simulink model "SpringiLQR3discrete"  (R2020b)
settings: Solver=FixedStepDiscrete  StartTime=0.0  StopTime=100  FixedStep=0.001  RelTol=1e-3
values from neighbouring files (symbols this model uses):
  A_e = full(kron(Ad, speye(2)))    [SringiLQR2discrete.m]    (also in SringiLQR3discrete.m; mpcgains.m = eye(n1+m1,n1+m1))
  B_e = full(kron(Bd, speye(2)))    [SringiLQR2discrete.m]    (also in SringiLQR3discrete.m; mpcgains.m = zeros(n1+m1,n_in))
  C_e = eye(4)    [SringiLQR2discrete.m]    (also in SringiLQR3discrete.m; mpcgains.m = zeros(m1,n1+m1))
  D_e = zeros(c1,b2)    [SringiLQR2discrete.m]    (also in SringiLQR3discrete.m)
  Dd = 0    [extmodel.m]
  Q = [1 0 0; 0 1 0; 0 0 10]    [LQR.m]    (also in NonlinearVehicleLQR.m = eye(3)*10; NonlinearVehicleiLQR.m = eye(3)*10; SringiLQR.m = [1 0; 0 1]*1; SringiLQR2.m = [1 0; 0 1]*1)
  Qf = eye(3)    [LQR.m]    (also in NonlinearVehicleLQR.m; NonlinearVehicleiLQR.m; SringiLQR.m = [1 0; 0 1]; SringiLQR2.m = [1 0; 0 1])
  R = eye(2)*10^-4    [LQR.m]    (also in NonlinearVehicleLQR.m = eye(2)*10^-2; NonlinearVehicleiLQR.m = eye(2)*10^-2; SringiLQR.m = eye(1)*1e-2; SringiLQR2.m = eye(1)*1e-2)
undefined symbols (not defined in the file or in its folder): Ad, Bd, Cd
libraries: pid_lib x1
settings Model: Creator=iris  LastModifiedBy=iris
settings DebuggingCC: SFMachineParentedDataDiag=error

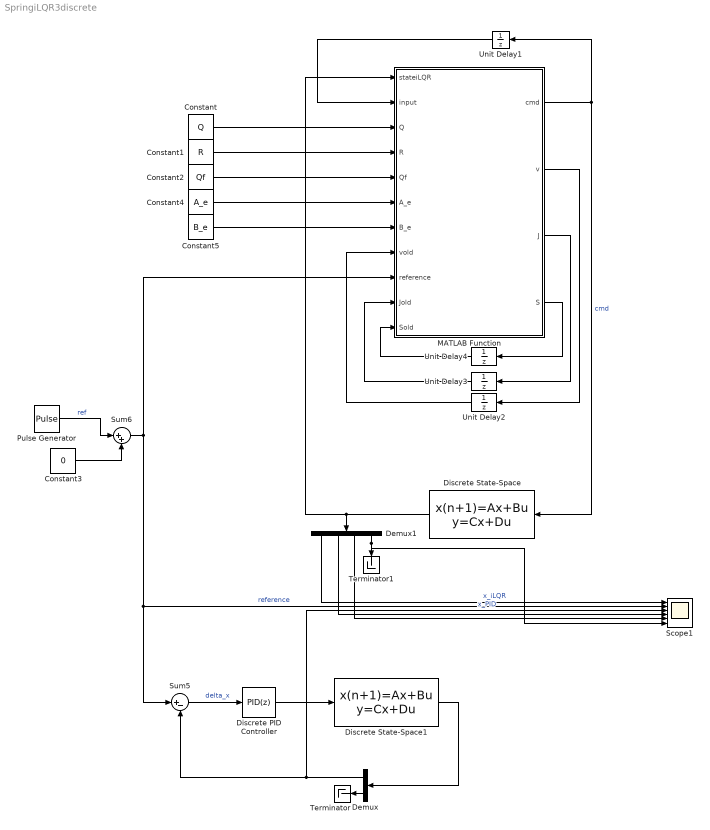
== system SpringiLQR3discrete ==
  Constant : Constant  Value=Q
  Constant1 : Constant  Value=R
  Constant2 : Constant  Value=Qf
  Constant3 : Constant  Value=0
  Constant4 : Constant  Value=A_e
  Constant5 : Constant  Value=B_e
  Demux : Demux  Outputs=2
  Demux1 : Demux
  Discrete PID Controller : pid_lib/PID Controller  Controller=PID  Form=Parallel  TimeDomain=Discrete-time  UseExternalTs=off  SampleTime=-1  IntegratorMethod=Forward Euler  FilterMethod=Forward Euler  ControllerParametersSource=internal  P=0.1  I=0  D=1  UseFilter=on  N=100  TunerSelectOption=Transfer Function Based (PID Tuner App)  InitialConditionSource=internal  InitialConditionForIntegrator=0  InitialConditionForFilter=0  DifferentiatorICPrevScaledInput=0  ExternalReset=none  TrackingMode=off  Kt=1  LimitOutput=off  SatLimitsSource=internal  UpperSaturationLimit=inf  LowerSaturationLimit=-inf  LinearizeAsGain=off  AntiWindupMode=none  Kb=1  POutMin=[]  POutMax=[]  IOutMin=[]  IOutMax=[]  DOutMin=[]  DOutMax=[]  NOutMin=[]  NOutMax=[]  SumOutMin=[]  SumOutMax=[]  SaturationOutMin=[]  SaturationOutMax=[]  PParamMin=[]  PParamMax=[]  IParamMin=[]  IParamMax=[]  DParamMin=[]  DParamMax=[]  NParamMin=[]  NParamMax=[]  KbParamMin=[]  KbParamMax=[]  KtParamMin=[]  KtParamMax=[]  KbOutMin=[]  KbOutMax=[]  KtOutMin=[]  KtOutMax=[]  IntegratorOutMin=[]  IntegratorOutMax=[]  FilterOutMin=[]  FilterOutMax=[]  SumI1OutMin=[]  SumI1OutMax=[]  SumI2OutMin=[]  SumI2OutMax=[]  SumI3OutMin=[]  SumI3OutMax=[]  SumI4OutMin=[]  SumI4OutMax=[]  SumDOutMin=[]  SumDOutMax=[]  DifferentiatorOutMin=[]  DifferentiatorOutMax=[]  FilterDiffOutCoefMin=[]  FilterDiffOutCoefMax=[]  ReciprocalOutMin=[]  ReciprocalOutMax=[]  SumDenOutMin=[]  SumDenOutMax=[]  SumNumOutMin=[]  SumNumOutMax=[]  DivideOutMin=[]  DivideOutMax=[]  UdiffTsProdOutMin=[]  UdiffTsProdOutMax=[]  NTsProdOutMin=[]  NTsProdOutMax=[]  UintegralTsProdOutMin=[]  UintegralTsProdOutMax=[]  UngainTsProdOutMin=[]  UngainTsProdOutMax=[]  IntegratorContinuousStateAttributes=''  IntegratorStateMustResolveToSignalObject=off  IntegratorRTWStateStorageClass=Auto  FilterContinuousStateAttributes=''  FilterStateMustResolveToSignalObject=off  FilterRTWStateStorageClass=Auto  ParallelPVariant=InternalParameters  IdealPVariant=Disabled  IVariant=InternalParameters  DVariant=InternalParameters  IntegratorVariant=Discrete  SatVariant=Disabled  AWVariant=Passthrough  PCopyVariant=Disabled  TRVariant=Disabled  FdbkBlocksVariant=Forward  IdealPFdbkVariant=Disabled  SatFdbkVariant=Disabled  DerivativeFilterVariant=ForwardEulerFilter  NVariant=InternalParameters  NCopyVariant=Disabled  FilterICVariant=InternalICsFilter  IntegratorICVariant=InternalICs  ExternalResetVariant=Disabled  TRSumVariant=Passthrough  SumFdbkVariant=Disabled  SumVariant=Sum_PID  TsampFilterVariant=InternalTs  TsampNgainVariant=Passthrough  TsampIntegralVariant=Passthrough  ExternalSaturationOutDataTypeStr=Inherit: Same as second input
  Discrete State-Space : DiscreteStateSpace  A=A_e  B=B_e  C=C_e  D=D_e  SampleTime=-1
  Discrete State-Space1 : DiscreteStateSpace  A=Ad  B=Bd  C=Cd  D=Dd  SampleTime=-1
  MATLAB Function : MATLAB Function  TreatAsAtomicUnit=on
  Pulse Generator : DiscretePulseGenerator  PulseType=Time based  Period=20  PulseWidth=50
  Scope1 : Scope  NumInputPorts=6
  Sum5 : Sum  Inputs=|+-
  Sum6 : Sum  Inputs=|++
  Terminator : Terminator
  Terminator1 : Terminator
  Unit Delay1 : UnitDelay  InitialCondition=zeros(1,2)  SampleTime=-1  HasFrameUpgradeWarning=on
  Unit Delay2 : UnitDelay  InitialCondition=ones(4,1)  SampleTime=-1  HasFrameUpgradeWarning=on
  Unit Delay3 : UnitDelay  InitialCondition=10000  SampleTime=-1  HasFrameUpgradeWarning=on
  Unit Delay4 : UnitDelay  InitialCondition=Qf  SampleTime=-1  HasFrameUpgradeWarning=on
  wires:
  Pulse Generator/1 -> Sum6/1  "ref"
  MATLAB Function/3(J) -> Unit Delay3/1
  MATLAB Function/2(v) -> Unit Delay2/1
  Constant/1 -> MATLAB Function/3(Q)
  Constant2/1 -> MATLAB Function/5(Qf)
  Constant1/1 -> MATLAB Function/4(R)
  MATLAB Function/1(cmd) -> Unit Delay1/1, Discrete State-Space/1  "cmd"
  Unit Delay2/1 -> MATLAB Function/8(vold)
  Sum5/1 -> Discrete PID Controller/1  "delta_x"
  Constant3/1 -> Sum6/2
  Sum6/1 -> MATLAB Function/9(reference), Sum5/1, Scope1/2  "reference"
  Unit Delay1/1 -> MATLAB Function/2(input)
  Unit Delay3/1 -> MATLAB Function/10(Jold)
  MATLAB Function/4(S) -> Unit Delay4/1
  Unit Delay4/1 -> MATLAB Function/11(Sold)
  Discrete State-Space1/1 -> Demux/1
  Demux/1 -> Sum5/2, Scope1/3  "x_PID"
  Demux/2 -> Terminator/1
  Discrete State-Space/1 -> Demux1/1, MATLAB Function/1(stateiLQR)
  Demux1/1 -> Scope1/1  "x_iLQR"
  Demux1/2 -> Scope1/4
  Constant4/1 -> MATLAB Function/6(A_e)
  Constant5/1 -> MATLAB Function/7(B_e)
  Discrete PID Controller/1 -> Discrete State-Space1/1
  Demux1/3 -> Scope1/5
  Demux1/4 -> Scope1/6, Terminator1/1

== matlab function SpringiLQR3discrete/MATLAB Function ==
  data: stateiLQR input; input input; Q input; R input; Qf input; A_e input; B_e input; vold input; reference input; cmd output; Jold input; Sold input; v output; J output; S output
function [cmd, v, J, S]= fcn(stateiLQR, input, Q, R, Qf, A_e, B_e, vold, reference, Jold, Sold)

% toll = 3*10^-5;

A = A_e;
B = B_e;
state = stateiLQR';
J = state*Qf*state'+state*Q*state'+input'*R*input;


% if abs(Jold-J)/Jold > toll
K  = (B'*Sold*B+R)\B'*Sold*A;
Kv = (B'*Sold*B+R)\B';
Ku = (B'*Sold*B+R)\R;
S  = A'*Sold*(A-B*K)+Q;
deltax = ones(size(K,2),1)*reference;
v  = (A-B*K)'*vold+Q*deltax-K'*R*input;
deltau = -K*state'-Kv*v-Ku*input;
cmd  = input + deltau;

% else
%     S  = Sold;
%     v  = vold;
%     cmd  = input';



end
